simulink model "DAQ_DB_Read_Test"  (Simulink 4.00)
settings: Solver=FixedStepDiscrete  StartTime=0.0  StopTime=inf  FixedStep=0.05  RelTol=1e-3
undefined symbols (not defined in the file or in its folder): gain, inputmode, polarity
settings Model: LastModifiedBy=bsaunder

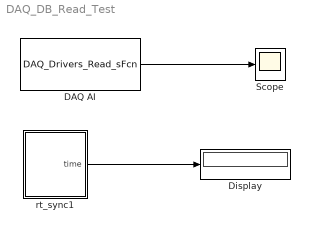
== system DAQ_DB_Read_Test ==
  DAQ AI : S-Function  FunctionName=DAQ_Drivers_Read_sFcn  Parameters=Ts, (inputmode-1), (polarity-1), gain, (channels-1)  PortCounts=[]  SFunctionModules=''  mask(DAQ_DB){channels=[1 2 3 4], gains=[1 1 1 1], scanTB_chbx=100 kHz (10 µs), scanInt=2, Ts=0.05}
      mask prompts: scanTB_chbx "Scan Timebase"; scanInt "Scan Interval"; Ts "Sample time"
      mask init:
      | if scanTB_chbx == 1 scanTB_chbx-1; end;
      | scanTB = scanTB_chbx-3;
      mask StyleString: edit,edit,popup(20 MHz (50 ns)|5 MHz (200 ns)|External|1 MHz (1µs)|100 kHz (10 µs)|10 kHz (100 µs)|1 kHz (1 ms)|100 Hz (10 ms)),edit,edit
  Display : Display
      settings: Format=short
  Scope : Scope
      settings: TimeRange=60  YMin=-5  YMax=5  SaveToWorkspace=off  SaveName=ScopeData  LimitDataPoints=on  MaxDataPoints=5000
  rt_sync1 : Subsystem  mask{Ts=0.05}
      mask prompts: Ts "Sample Time"
      settings: RTWFcnNameOpts=Auto  RTWFileNameOpts=Auto
      mask Display: fprintf('Real\n Time\n sync')
  wires:
  DAQ AI/1 -> Scope/1
  rt_sync1/1(time) -> Display/1

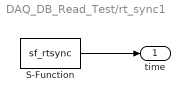
== system DAQ_DB_Read_Test/rt_sync1 ==
  S-Function : S-Function  FunctionName=sf_rtsync  Parameters=Ts  PortCounts=[]  SFunctionModules=''
  time : Outport  Port=1
  wires:
  S-Function/1 -> time/1
